simulink model "MCU_M"  (R2023a)
settings: Solver=VariableStepAuto  StartTime=0.0  StopTime=10.0  RelTol=1e-3
settings Model: Creator=romav  LastModifiedBy=romav
settings DataIOCC: SaveOutput=off  SaveTime=off

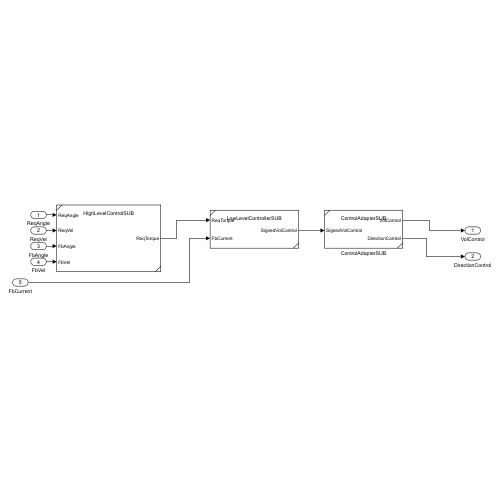
[thumbnail: Simulink's stored preview of the top-level diagram]
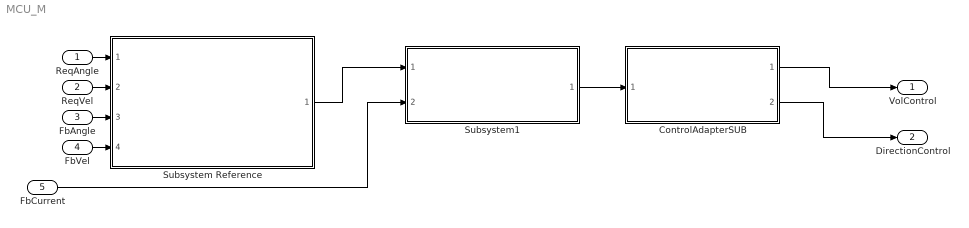
== system MCU_M ==
  ReqAngle : Inport  OutDataTypeStr=double  PortDimensions=1
  ReqVel : Inport  Port=2  OutDataTypeStr=double  PortDimensions=1
  FbAngle : Inport  Port=3  OutDataTypeStr=double  PortDimensions=1
  FbVel : Inport  Port=4  OutDataTypeStr=double  PortDimensions=1
  FbCurrent : Inport  Port=5  OutDataTypeStr=double  PortDimensions=1  SampleTime=0
  ControlAdapterSUB : Subsystem  ReferencedSubsystem=ControlAdapterSUB
  Subsystem Reference : Subsystem  ReferencedSubsystem=HighLevelControlSUB
  Subsystem1 : Subsystem  ReferencedSubsystem=LowLevelControllerSUB
  VolControl : Outport  OutDataTypeStr=double  PortDimensions=1  SampleTime=0
  DirectionControl : Outport  Port=2  OutDataTypeStr=double  PortDimensions=1  SampleTime=0
  wires:
  ReqAngle/1 -> Subsystem Reference/1
  FbAngle/1 -> Subsystem Reference/3
  ReqVel/1 -> Subsystem Reference/2
  Subsystem1/1 -> ControlAdapterSUB/1
  Subsystem Reference/1 -> Subsystem1/1
  FbVel/1 -> Subsystem Reference/4
  ControlAdapterSUB/1 -> VolControl/1
  FbCurrent/1 -> Subsystem1/2
  ControlAdapterSUB/2 -> DirectionControl/1
